simulink model "CoffeeReactor_task31"  (R2023b)
settings: Solver=ode4  StartTime=0.0  StopTime=simulationParameters.Tsim  FixedStep=simulationParameters.Tint  RelTol=1e-3
undefined symbols (not defined in the file): compute_MPC_control, condensedMatrices, m_input, n, p, PH, simulationParameters, sys_d, u_0
settings Model: Creator=simone  LastModifiedBy=viola
settings SolverCC: AlgebraicLoopSolver=TrustRegion
settings DataIOCC: SaveOutput=off  SignalLogging=off  DSMLogging=off  SaveTime=off  ReturnWorkspaceOutputs=off
settings DebuggingCC: UnconnectedInputMsg=warning  UnconnectedOutputMsg=warning  UnconnectedLineMsg=warning
settings ModelReferenceCC: EnableRefExpFcnMdlSchedulingChecks=on
settings RTWCC: DLArmComputeVersion=19.05

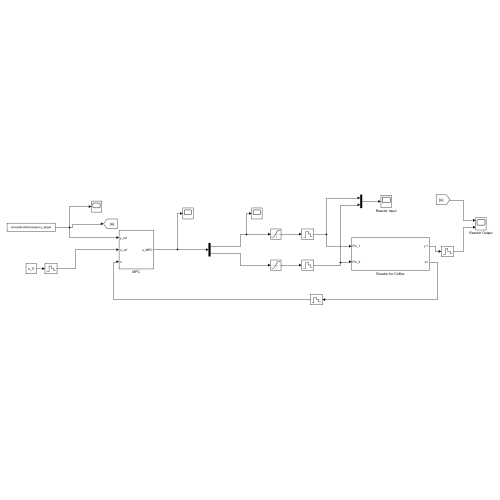
[thumbnail: Simulink's stored preview of the top-level diagram]
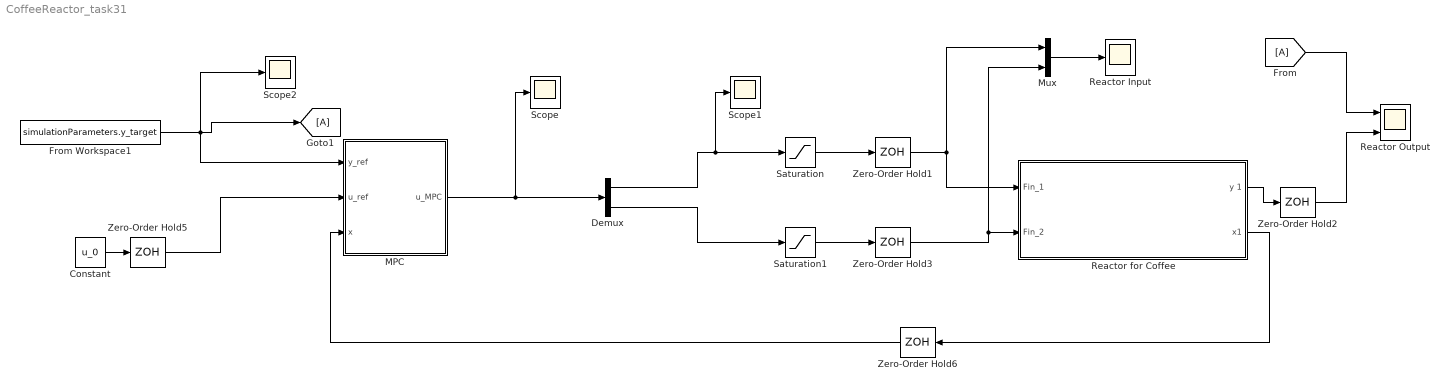
== system CoffeeReactor_task31 ==
  Constant : Constant  Value=u_0
  Demux : Demux  Outputs=2
  From : From
  From Workspace1 : FromWorkspace  VariableName=simulationParameters.y_target  OutputAfterFinalValue=Holding final value
  Goto1 : Goto
  MPC : Subsystem
  Mux : Mux  Inputs=2
  Reactor Input : Scope
  Reactor Output : Scope  NumInputPorts=2
  Reactor for Coffee : Subsystem
  Saturation : Saturate  UpperLimit=simulationParameters.Fin1_max  LowerLimit=simulationParameters.Fin1_min
  Saturation1 : Saturate  UpperLimit=simulationParameters.Fin2_max  LowerLimit=simulationParameters.Fin2_min
  Scope : Scope
  Scope1 : Scope
  Scope2 : Scope
  Zero-Order Hold{1..3,5..6} (5 alike) : ZeroOrderHold  SampleTime=simulationParameters.Ts
  wires:
  Zero-Order Hold2/1 -> Reactor Output/2
  From/1 -> Reactor Output/1
  Mux/1 -> Reactor Input/1
  Zero-Order Hold1/1 -> Reactor for Coffee/1(Fin_1), Mux/1
  Zero-Order Hold3/1 -> Mux/2, Reactor for Coffee/2(Fin_2)
  Saturation/1 -> Zero-Order Hold1/1
  Saturation1/1 -> Zero-Order Hold3/1
  Zero-Order Hold5/1 -> MPC/2(u_ref)
  Constant/1 -> Zero-Order Hold5/1
  MPC/1(u_MPC) -> Scope/1, Demux/1
  Demux/1 -> Scope1/1, Saturation/1
  Demux/2 -> Saturation1/1
  Reactor for Coffee/1(y 1) -> Zero-Order Hold2/1
  Reactor for Coffee/2(x1) -> Zero-Order Hold6/1
  Zero-Order Hold6/1 -> MPC/3(x)
  From Workspace1/1 -> MPC/1(y_ref), Goto1/1, Scope2/1

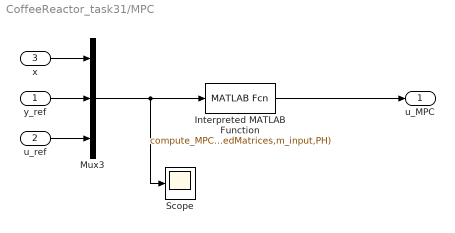
== system CoffeeReactor_task31/MPC ==
  y_ref : Inport
  u_ref : Inport  Port=2
  x : Inport  Port=3
  Interpreted MATLAB Function : MATLABFcn  MATLABFcn=compute_MPC_control(u(1:n),u(n+1:n+p),u(n+p+1:n+p+m_input),condensedMatrices,m_input,PH)  OutputDimensions=m_input  Output1D=off
  Mux3 : Mux  Inputs=3
  Scope : Scope
  u_MPC : Outport
  wires:
  Interpreted MATLAB Function/1 -> u_MPC/1
  x/1 -> Mux3/1
  y_ref/1 -> Mux3/2
  Mux3/1 -> Scope/1, Interpreted MATLAB Function/1
  u_ref/1 -> Mux3/3

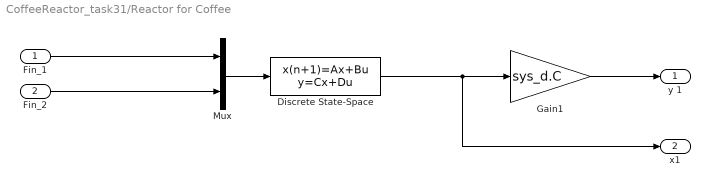
== system CoffeeReactor_task31/Reactor for Coffee ==
  Fin_1 : Inport
  Fin_2 : Inport  Port=2
  Discrete State-Space : DiscreteStateSpace  A=sys_d.A  B=sys_d.B  C=sys_d.C  D=sys_d.D  InitialCondition=simulationParameters.Reactor_parameters.x_0  SampleTime=-1
  Gain1 : Gain  Gain=sys_d.C
  Mux : Mux  Inputs=2
  y 1 : Outport
  x1 : Outport  Port=2
  wires:
  Fin_2/1 -> Mux/2
  Fin_1/1 -> Mux/1
  Mux/1 -> Discrete State-Space/1
  Discrete State-Space/1 -> Gain1/1, x1/1
  Gain1/1 -> y 1/1
